simulink model "DBX_model_all"  (R2015a)
settings: Solver=ode2  SolverMode=SingleTasking  StartTime=0.0  StopTime=10  FixedStep=T_sim  RelTol=1e-3
undefined symbols (not defined in the file): A_M, Alpha_unique_rad, as, B_span, Beta_unique_rad, C_D_q, C_l, C_l_delta_a_Asim, C_l_delta_rv_Asim, C_l_p, C_l_r, C_Lift_q, C_m, C_m_q, C_n, C_n_delta_a_Asim, C_n_delta_rv_Asim, C_n_p, C_n_r, C_X, C_Y, C_Y_delta_rv_Asim, C_Y_p, C_Y_r, C_Z, CG, CMA, DBX_aero, DBX_aero_param, delta_elev_unique_rad, DOWN_0, EAST_0, F, g, h_1, h_2, h_3, I_BAC, Initial_Omegas, Initial_Torques, Ion, L_M, Lithium, m, MIL, NORTH_0, P_0, Q_0, R_0, Rotation_sign, Servo_calib, T_sim, U_0, V_0, W_0
libraries: simulink x19, DBX_model x14, aerolibwind2 x12, aerolibasang x9, aerolibadyn x4, aerolibatmos2 x2, powerlib x2, aerolibtransform2 x1, electricdrivelib x1
(part 1 of 3)
settings Model: ExtModeTrigDuration=5000  Creator=DavidTorres  LastModifiedBy=David
settings DataIOCC: LimitDataPoints=off  SaveOutput=off  SignalLogging=off  DSMLogging=off  VisualizeSimOutput=off  SaveTime=off
settings OptimizationCC: InlineParams=on  UseDivisionForNetSlopeComputation=on  UseFloatMulNetSlope=on  InlineInvariantSignals=on  EnhancedBackFolding=on  EfficientFloat2IntCast=on  SimCompilerOptimization=on
settings DebuggingCC: AlgebraicLoopMsg=error  ArtificialAlgebraicLoopMsg=error  SaveWithParameterizedLinksMsg=none  UniqueDataStoreMsg=error  StrictBusMsg=ErrorOnBusTreatedAsVector
settings HardwareCC: ProdLargestAtomicInteger=Long  ProdLargestAtomicFloat=Float  ProdIntDivRoundTo=Zero  ProdEndianess=LittleEndian  ProdHWDeviceType=ARM Compatible->ARM 7  TargetUnknown=on
settings ModelReferenceCC: ModelReferenceNumInstancesAllowed=Single  ModelReferencePassRootInputsByReference=off
settings SimscapeCC: EditingMode=Restricted

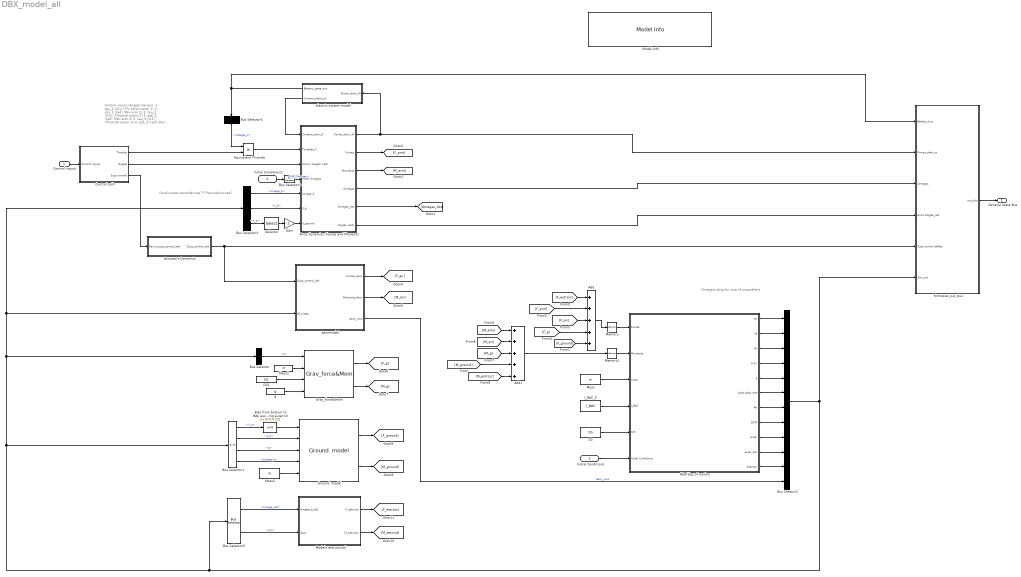
== system DBX_model_all ==
  note: Condiciones atmosfericas???
      | Perturbaciones?
  note: Omegas=Angular rate of proppellers
  note: Control inputs (Angles Servos):
      |
      | 1. tau_1 [0-1] (Thr ottle motor 1)
      | 2. eta_1 (rad)  (Pan arm 1)
      |
      | 3. tau_2 [0-1] (Throttle motor 2)
      | 4. eta_2 (rad)  (Pan arm 2)
      |
      | 5. tau_3 [0-1] (Throttle motor 3)
      | 6. eta_3 (rad)  (Pan arm  3)
      |
      | 7. Rudervator Left (rad)
      | 8. Rudervator Right (rad)
      | 9. Aileron Left (rad)
      | 10. Aielron Right (rad)
  Control Inputs : Inport  PortDimensions=[10,1]
  Initial Conditions : Inport  Port=2  OutDataTypeStr=Bus: slBus1
  6dof Eqs of motion : Subsystem
  Actuators Dynamcis : Subsystem  TreatAsAtomicUnit=on
  Add : Sum  Inputs=+++++
  Add1 : Sum  Inputs=+++++
  Aeromodel : Subsystem  Variant=on  OverrideUsingVariant=DBX_aeroV2_param
  Arms Dynamics: Forces and Moments : Subsystem
  Bias from bottom to BAC assuming euler=0 : Bias  Bias=[0;0;0.25]
  Bus Creator1 : BusCreator  Inputs=12
  Bus Selector : BusSelector  OutputSignals=q
  Bus Selector1 : BusSelector  OutputSignals=X_e,V_b,q,omega_b
  Bus Selector2 : BusSelector  OutputSignals=omega_b,V_b,X_e
  Bus Selector3 : BusSelector  OutputSignals=Init_Omegas
  Bus Selector4 : BusSelector  OutputSignals=Voltage_V
  Bus Selector5 : BusSelector  OutputSignals=omega_dot,A_b
  CG : Constant  Value=CG
  CG1 : Constant  Value=CG
  Control split : Subsystem
  Equivalent Throttle : Product  Inputs=**
  Gain : Gain  Gain=-1
  Grav_force&Mom : DBX_model/Grav_force&Mom
  Ground  model : DBX_model/Ground  model
  I_BAC_0 : Constant  Value=I_BAC
  Initial Conditions1 : InportShadow  Port=2  OutDataTypeStr=Bus: slBus1
  Mass : Constant  Value=m
  Mass1 : Constant  Value=m
  Mass2 : Constant  Value=m
  Memory : Memory  X0=[0,0,0]'  InheritSampleTime=on
  Memory1 : Memory  X0=[0,0,0]'  InheritSampleTime=on
  Model Info : simulink/Model-Wide Utilities/Model Info  Frame=on  DisplayStringWithTags=|  HorizontalTextAlignment=Center  LeftAlignmentValue=0.5  SourceBlockDiagram=DBX_model_all  TagMaxNumber=20
      | Model %<ModelName>
      | 
      | Creado por %<Creator>
      | Modificado el %<LastModificationDate> por %<LastModifiedBy>
      | Version %<ModelVersion>
  Modelo estructural : Subsystem
  Selector : Selector  InputPortWidth=3  Indices=3
  electric system model : Subsystem
  formateo_out_bus : Subsystem
  "g " : Constant  Value=g
  General State Bus : Outport  OutDataTypeStr=Bus: slBus4
  wires:
  Initial Conditions/1 -> 6dof Eqs of motion/6(Initial Conditions)
  6dof Eqs of motion/3(Vb) -> Bus Creator1/3
  6dof Eqs of motion/5(q) -> Bus Creator1/5
  6dof Eqs of motion/2(Ve) -> Bus Creator1/2
  6dof Eqs of motion/6(pdot,qdot,rdot) -> Bus Creator1/6
  6dof Eqs of motion/1(Xe) -> Bus Creator1/1
  6dof Eqs of motion/7(Ab) -> Bus Creator1/7
  6dof Eqs of motion/8(DCM) -> Bus Creator1/8
  6dof Eqs of motion/9(euler) -> Bus Creator1/9
  6dof Eqs of motion/10(euler_dot) -> Bus Creator1/10
  Bus Selector/1 -> Grav_force&Mom/1  "<q>"
  Mass/1 -> 6dof Eqs of motion/3(mass)
  Bus Selector2/1 -> Arms Dynamics: Forces and Moments/5(omega_b)  "<omega_b>"
  Bus Selector2/2 -> Arms Dynamics: Forces and Moments/6(V_b)  "<V_b>"
  Mass1/1 -> Grav_force&Mom/2
  Arms Dynamics: Forces and Moments/5(Omegas_dot) -> [Omegas_dot]
  Initial Conditions1/1 -> Bus Selector3/1
  Bus Selector2/3 -> Selector/1  "<X_e>"
  Selector/1 -> Gain/1
  Gain/1 -> Arms Dynamics: Forces and Moments/7(h_ground)
  Arms Dynamics: Forces and Moments/2(Forces) -> [F_arm]
  Arms Dynamics: Forces and Moments/3(Moments) -> [M_arm]
  Grav_force&Mom/1 -> [F_g]
  [F_arm] -> Add/2
  [F_air] -> Add/3
  [F_g] -> Add/4
  [M_arm] -> Add1/1
  [M_g] -> Add1/3
  [M_air] -> Add1/2
  6dof Eqs of motion/11(Asensor) -> Bus Creator1/11
  Control split/1("Throtles ") -> Equivalent Throttle/2
  Control split/2(Angles) -> Arms Dynamics: Forces and Moments/3(Comm Angles (rad))
  Arms Dynamics: Forces and Moments/4(Omegas) -> formateo_out_bus/3(Omegas)
  Memory/1 -> 6dof Eqs of motion/1(Forces)
  Memory1/1 -> 6dof Eqs of motion/2(Moments)
  CG/1 -> 6dof Eqs of motion/5(CG)
  I_BAC_0/1 -> 6dof Eqs of motion/4(I_BAC)
  Equivalent Throttle/1 -> Arms Dynamics: Forces and Moments/2(Throttles_V)
  Bus Selector4/1 -> Equivalent Throttle/1  "<Voltage_V>"
  6dof Eqs of motion/4(p,q,r) -> Bus Creator1/4
  Arms Dynamics: Forces and Moments/6(Angles (rad)) -> formateo_out_bus/4(Arms Angles_rad)
  Control Inputs/1 -> Control split/1(Control inputs)
  CG1/1 -> Grav_force&Mom/3
  Control split/3(Sups control) -> Actuators Dynamcis/1(Servo_sups_control_rad)
  formateo_out_bus/1(out_bus) -> General State Bus/1
  Bus Selector3/1 -> Arms Dynamics: Forces and Moments/4(Initial Omegas)  "<Init_Omegas>"
  Actuators Dynamcis/1(Sups_control_rad) -> Aeromodel/1(Sups_control_rad), formateo_out_bus/5(Sups control deflec)
  Add/1 -> Memory/1
  Aeromodel/3(Aero_vars) -> Bus Creator1/12  "Aero_vars"
  Add1/1 -> Memory1/1
  Aeromodel/1(Forces_aero) -> [F_air]
  Bus Creator1/1 -> formateo_out_bus/6(Sim_out), Bus Selector5/1, Bus Selector/1, Bus Selector2/1, Aeromodel/2(All_meas), Bus Selector1/1
  Ground  model/1 -> [F_ground]
  Ground  model/2 -> [M_ground]
  Bus Selector1/1 -> Bias from bottom to BAC assuming euler=0/1  "<X_e>"
  Bus Selector1/3 -> Ground  model/3  "<q>"
  Mass2/1 -> Ground  model/5
  Bus Selector1/2 -> Ground  model/2  "<V_b>"
  Bus Selector1/4 -> Ground  model/4  "<omega_b>"
  Bias from bottom to BAC assuming euler=0/1 -> Ground  model/1
  "g "/1 -> Grav_force&Mom/4
  [M_ground] -> Add1/4
  [F_ground] -> Add/5
  Aeromodel/2(Moments_Aero) -> [M_air]
  electric system model/1(Battery_state_bus) -> Bus Selector4/1, formateo_out_bus/1(Battery_bus)
  Arms Dynamics: Forces and Moments/1(Power_drain_W) -> electric system model/1(Power_drain_W), formateo_out_bus/2(Power_drain_w)
  electric system model/2(Current_drains_A) -> Arms Dynamics: Forces and Moments/1(Current_drain_A)
  Bus Selector5/1 -> Modelo estructural/1(omgea_b_dot)  "<omega_dot>"
  Modelo estructural/2(M_estructu) -> [M_estrcut]
  [M_estrcut] -> Add1/5
  Bus Selector5/2 -> Modelo estructural/2(Accs)  "<A_b>"
  Modelo estructural/1(F_estructu) -> [F_estrcut]
  [F_estrcut] -> Add/1
  Grav_force&Mom/2 -> [M_g]

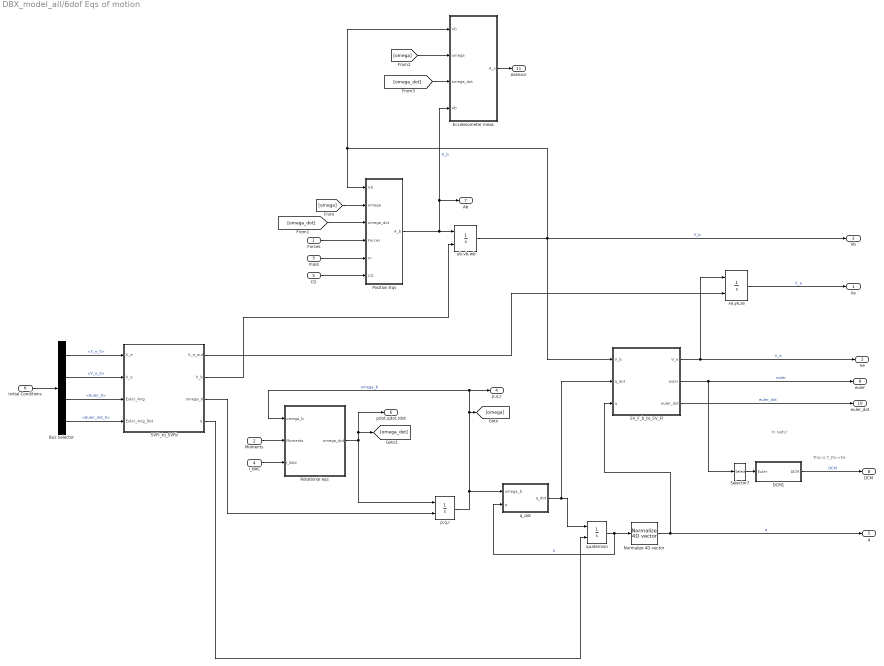
== system DBX_model_all/6dof Eqs of motion ==
  note: In rads!
  note: This is T_Fb->Fe
  Forces : Inport
  Moments : Inport  Port=2
  mass : Inport  Port=3
  I_BAC : Inport  Port=4
  CG : Inport  Port=5
  Initial Conditions : Inport  Port=6
  Bus Selector : BusSelector  OutputSignals=X_e_0,V_e_0,Euler_0,Euler_dot_0
  DCM1 : Subsystem  TreatAsAtomicUnit=on
  Eccelerometer meas : MATLAB Function
  Normalize 4D vector : DBX_model/Normalize 4D vector
  Position Eqs : MATLAB Function
  Rotational eqs : MATLAB Function
  SVFI_to_SVFb : MATLAB Function
  SV_F_b_to_SV_FI : MATLAB Function
  Selector7 : Selector  InputPortWidth=3  Indices=[3 2 1]
  "p,q,r " : Integrator  InitialConditionSource=external  InitialCondition=[P_0,Q_0,R_0]
  q_dot : Subsystem
  quaternion : Integrator  InitialConditionSource=external  InitialCondition=[P_0,Q_0,R_0]
  ub,vb,wb : Integrator  InitialConditionSource=external  InitialCondition=[U_0,V_0,W_0]
  xe,ye,ze : Integrator  InitialConditionSource=external  InitialCondition=[NORTH_0,EAST_0,-DOWN_0]
  Xe : Outport
  Ve : Outport  Port=2
  Vb : Outport  Port=3
  p,q,r : Outport  Port=4
  q : Outport  Port=5
  pdot,qdot,rdot : Outport  Port=6
  Ab : Outport  Port=7
  DCM : Outport  Port=8
  euler : Outport  Port=9
  euler_dot : Outport  Port=10
  Asensor : Outport  Port=11
  wires:
  I_BAC/1 -> Rotational eqs/3(I_BAC)
  mass/1 -> Position Eqs/5(m)
  Forces/1 -> Position Eqs/4(Forces)
  xe,ye,ze/1 -> Xe/1  "X_e"
  ub,vb,wb/1 -> Eccelerometer meas/1(Vb), Position Eqs/1(Vb), Vb/1, SV_F_b_to_SV_FI/1(V_b)  "V_b"
  SV_F_b_to_SV_FI/1(V_e) -> Ve/1, xe,ye,ze/1  "V_e"
  [omega] -> Position Eqs/2(omega)
  [omega_dot] -> Position Eqs/3(omega_dot)
  Position Eqs/1(A_b) -> Eccelerometer meas/4(Ab), Ab/1, ub,vb,wb/1  "A_b"
  CG/1 -> Position Eqs/6(CG)
  Initial Conditions/1 -> Bus Selector/1
  Bus Selector/1 -> SVFI_to_SVFb/1(X_e)  "<X_e_0>"
  Bus Selector/2 -> SVFI_to_SVFb/2(V_e)  "<V_e_0>"
  Bus Selector/3 -> SVFI_to_SVFb/3(Euler_Ang)  "<Euler_0>"
  Bus Selector/4 -> SVFI_to_SVFb/4(Euler_Ang_Dot)  "<Euler_dot_0>"
  SVFI_to_SVFb/2(V_b) -> ub,vb,wb/2
  SVFI_to_SVFb/1(X_e_out) -> xe,ye,ze/2
  SVFI_to_SVFb/3(omega_b) -> "p,q,r "/2
  "p,q,r "/1 -> q_dot/1(omega_b), Rotational eqs/1(omega_b), p,q,r/1, [omega]  "omega_b"
  q_dot/1(q_dot) -> quaternion/1, SV_F_b_to_SV_FI/2(q_dot)
  SVFI_to_SVFb/4(q) -> quaternion/2
  quaternion/1 -> Normalize 4D vector/1, q_dot/2(q)  "q"
  DCM1/1(DCM) -> DCM/1  "DCM"
  SV_F_b_to_SV_FI/3(euler_dot) -> euler_dot/1  "euler_dot"
  Moments/1 -> Rotational eqs/2(Moments)
  Normalize 4D vector/1 -> q/1, SV_F_b_to_SV_FI/3(q)  "q"
  [omega] -> Eccelerometer meas/2(omega)
  [omega_dot] -> Eccelerometer meas/3(omega_dot)
  Eccelerometer meas/1(A_s) -> Asensor/1
  Selector7/1 -> DCM1/1(Euler)
  Rotational eqs/1(omega_dot) -> "p,q,r "/1, pdot,qdot,rdot/1, [omega_dot]
  SV_F_b_to_SV_FI/2(euler) -> Selector7/1, euler/1  "euler"

== system DBX_model_all/Actuators Dynamcis ==
  note: Relaciones no lineales aqui
  note: Control inputs:
      |
      |
      | 7. Rudervator Left (rad)
      | 8. Rudervator Right (rad)
      | 9. Aileron Left (rad)
      | 10. Aielron Right (rad)
  Servo_sups_control_rad : Inport
  Demux : Demux
  Mux2 : Mux
  Servo 1st order : DBX_model/Servo 1st order  Init_def=delta_rv_L_0_servo  Max_rate=6.159  Min_rate=-6.159  Max_defle=deg2rad(25)  Min_def=-deg2rad(25)  RT=0.01
  Servo 1st order1 : DBX_model/Servo 1st order  Init_def=delta_rv_R_0_servo  Max_rate=6.159  Min_rate=-6.159  Max_defle=deg2rad(25)  Min_def=-deg2rad(25)  RT=0.01
  Servo 1st order2 : DBX_model/Servo 1st order  Init_def=delta_a_L_0_servo  Max_rate=6.159  Min_rate=-6.159  Max_defle=deg2rad(25)  Min_def=-deg2rad(25)  RT=0.01
  Servo 1st order3 : DBX_model/Servo 1st order  Init_def=delta_a_R_0_servo  Max_rate=6.159  Min_rate=-6.159  Max_defle=deg2rad(25)  Min_def=-deg2rad(25)  RT=0.01
  Servo2Sup Lin conversion : DBX_model/Servo2Sup Lin conversion  Gain=Servo_calib.Servo4.Pendiente_Sup_Servo  Bias=Servo_calib.Servo4.Sup_rad_0
  Servo2Sup Lin conversion1 : DBX_model/Servo2Sup Lin conversion  Gain=Servo_calib.Servo5.Pendiente_Sup_Servo  Bias=Servo_calib.Servo5.Sup_rad_0
  Servo2Sup Lin conversion2 : DBX_model/Servo2Sup Lin conversion  Gain=Servo_calib.Servo6.Pendiente_Sup_Servo  Bias=Servo_calib.Servo6.Sup_rad_0
  Servo2Sup Lin conversion3 : DBX_model/Servo2Sup Lin conversion  Gain=Servo_calib.Servo7.Pendiente_Sup_Servo  Bias=Servo_calib.Servo7.Sup_rad_0
  Sups_control_rad : Outport
  wires:
  Servo_sups_control_rad/1 -> Demux/1
  Mux2/1 -> Sups_control_rad/1
  Demux/1 -> Servo 1st order/1
  Demux/2 -> Servo 1st order1/1
  Demux/3 -> Servo 1st order2/1
  Demux/4 -> Servo 1st order3/1
  Servo2Sup Lin conversion/1 -> Mux2/1
  Servo2Sup Lin conversion1/1 -> Mux2/2
  Servo2Sup Lin conversion2/1 -> Mux2/3
  Servo2Sup Lin conversion3/1 -> Mux2/4
  Servo 1st order/1 -> Servo2Sup Lin conversion/1
  Servo 1st order1/1 -> Servo2Sup Lin conversion1/1
  Servo 1st order2/1 -> Servo2Sup Lin conversion2/1
  Servo 1st order3/1 -> Servo2Sup Lin conversion3/1

== system DBX_model_all/Aeromodel ==
  note: 1) Add Subsystem or Model blocks as valid variant choices.
      | 2) You cannot connect blocks at this level. At simulation, connectivity is automatically
      | determined, based on the active variant and port name matching.
  Sups_control_rad : Inport
  All_meas : Inport  Port=2
  Aero model V1 : Subsystem  VariantControl=DBX_aeroV1
  Aero model V2 : Subsystem  VariantControl=DBX_aeroV2
  Aero model V2 parametric : Subsystem  VariantControl=DBX_aeroV2_param
  Aero model aerosonde : Subsystem  VariantControl=AeroAerosonde
  Forces_aero : Outport
  Moments_Aero : Outport  Port=2
  Aero_vars : Outport  Port=3

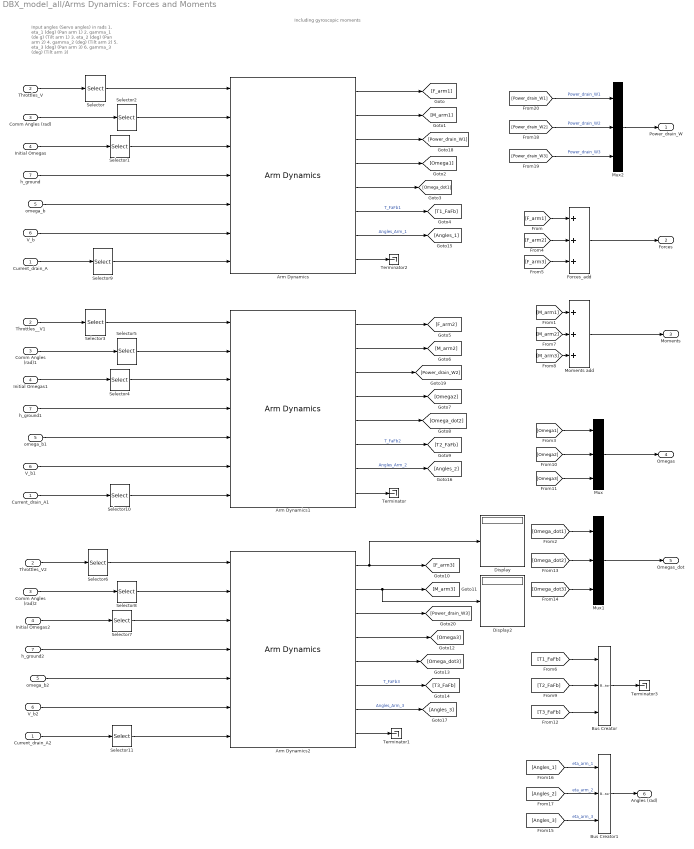
== system DBX_model_all/Arms Dynamics: Forces and Moments ==
  note: Including gyroscopic moments
  note: Input angles (Servo angles)  in rads
      |
      | 1. eta_1 (deg)  (Pan arm 1)
      | 2. gamma_1 (de g)  (Tilt arm 1)
      |
      | 3. eta_2 (deg)  (Pan arm 2)
      | 4. gamma_2 (deg)  (Tilt arm 2)
      |
      | 5. eta_3 (deg)  (Pan arm  3)
      | 6. gamma_3 (deg)  (Tilt arm 3)
  Current_drain_A : Inport
  Throttles_V : Inport  Port=2
  Comm Angles (rad) : Inport  Port=3
  Initial Omegas : Inport  Port=4
  omega_b : Inport  Port=5
  V_b : Inport  Port=6
  h_ground : Inport  Port=7
  Arm Dynamics : DBX_model/Arm Dynamics  arm_num=1  Rot_sign=Rotation_sign(1)  Hub_pos=[1/3*L_M;-A_M/2;h_1]  h_p=hp_1  Gain=[0;1;0]  UpperLimit=deg2rad(10)  LowerLimit=-deg2rad(90)  J_FA=J_FA_1  Inertia_swithc_var=None  Freno_param=Activo  J_T=J_T  tau=Tau_motors  Initi_omega=Initial_Omegas(1)  Init_torque=Initial_Torques(1)  omega_n=40  xi=1.45  init_eta=eta_1_0_servo  Gain_servos=Servo_calib.Servo1.Pendiente_Sup_Servo  Bias=Servo_calib.Servo1.Sup_rad_0
  Arm Dynamics1 : DBX_model/Arm Dynamics  arm_num=2  Rot_sign=Rotation_sign(2)  Hub_pos=[1/3*L_M;A_M/2;h_2]  h_p=hp_2  Gain=[0;1;0]  UpperLimit=deg2rad(10)  LowerLimit=-deg2rad(90)  J_FA=J_FA_2  Inertia_swithc_var=None  Freno_param=Activo  J_T=J_T  tau=Tau_motors  Initi_omega=Initial_Omegas(2)  Init_torque=Initial_Torques(2)  omega_n=40  xi=1.45  init_eta=eta_2_0_servo  Gain_servos=Servo_calib.Servo2.Pendiente_Sup_Servo  Bias=Servo_calib.Servo2.Sup_rad_0
  Arm Dynamics2 : DBX_model/Arm Dynamics  arm_num=3  Rot_sign=Rotation_sign(3)  Hub_pos=[-2/3*L_M;0;h_3]  h_p=hp_3  Gain=[1;0;0]  UpperLimit=deg2rad(60)  LowerLimit=-deg2rad(60)  J_FA=J_FA_3  Inertia_swithc_var=None  Freno_param=Activo  J_T=J_T  tau=Tau_motors  Initi_omega=Initial_Omegas(3)  Init_torque=Initial_Torques(3)  omega_n=40  xi=1.45  init_eta=eta_3_0  Gain_servos=Servo_calib.Servo3.Pendiente_Sup_Servo  Bias=Servo_calib.Servo3.Sup_rad_0
  Bus Creator : BusCreator  Inputs=3
  Bus Creator1 : BusCreator  Inputs=3
  Comm Angles (rad)1 : InportShadow  Port=3
  Comm Angles (rad)2 : InportShadow  Port=3
  Current_drain_A1 : InportShadow
  Current_drain_A2 : InportShadow
  Display : Display
  Display2 : Display
  Forces_add : Sum  Inputs=+++
  Initial Omegas1 : InportShadow  Port=4
  Initial Omegas2 : InportShadow  Port=4
  Moments add : Sum  Inputs=+++
  Mux : Mux  Inputs=3
  Mux1 : Mux  Inputs=3
  Mux2 : Mux  Inputs=3
  Selector : Selector  InputPortWidth=3  Indices=[1]
  Selector1 : Selector  InputPortWidth=3  Indices=[1]
  Selector{3..5,10} (4 alike) : Selector  InputPortWidth=3  Indices=2
  Selector{6..8,11} (4 alike) : Selector  InputPortWidth=3  Indices=3
  Selector2 : Selector  InputPortWidth=3
  Selector9 : Selector  InputPortWidth=3  Indices=[1]
  Terminator{,1..3} (4 alike) : Terminator
  Throttles_V2 : InportShadow  Port=2
  Throttles__V1 : InportShadow  Port=2
  V_b1 : InportShadow  Port=6
  V_b2 : InportShadow  Port=6
  h_ground1 : InportShadow  Port=7
  h_ground2 : InportShadow  Port=7
  omega_b1 : InportShadow  Port=5
  omega_b2 : InportShadow  Port=5
  Power_drain_W : Outport
  Forces : Outport  Port=2
  Moments : Outport  Port=3
  Omegas : Outport  Port=4
  Omegas_dot : Outport  Port=5
  Angles (rad) : Outport  Port=6
  wires:
  Selector1/1 -> Arm Dynamics/3
  Throttles_V/1 -> Selector/1
  Initial Omegas/1 -> Selector1/1
  Selector/1 -> Arm Dynamics/1
  V_b/1 -> Arm Dynamics/6
  Forces_add/1 -> Forces/1
  Moments add/1 -> Moments/1
  Mux/1 -> Omegas/1
  Mux1/1 -> Omegas_dot/1
  h_ground/1 -> Arm Dynamics/4
  Arm Dynamics/1 -> [F_arm1]
  Arm Dynamics/2 -> [M_arm1]
  Arm Dynamics/4 -> [Omega1]
  Arm Dynamics/5 -> [Omega_dot1]
  [F_arm1] -> Forces_add/1
  [M_arm1] -> Moments add/1
  [Omega_dot1] -> Mux1/1
  [Omega1] -> Mux/1
  omega_b/1 -> Arm Dynamics/5
  [F_arm2] -> Forces_add/2
  [F_arm3] -> Forces_add/3
  [Omega2] -> Mux/2
  [Omega3] -> Mux/3
  [Omega_dot2] -> Mux1/2
  [Omega_dot3] -> Mux1/3
  [M_arm3] -> Moments add/3
  [M_arm2] -> Moments add/2
  Selector2/1 -> Arm Dynamics/2
  Comm Angles (rad)/1 -> Selector2/1
  Arm Dynamics/6 -> [T1_FaFb]  "T_FaFb1"
  [T1_FaFb] -> Bus Creator/1
  Selector4/1 -> Arm Dynamics1/3
  Throttles__V1/1 -> Selector3/1
  Initial Omegas1/1 -> Selector4/1
  Selector3/1 -> Arm Dynamics1/1
  V_b1/1 -> Arm Dynamics1/6
  h_ground1/1 -> Arm Dynamics1/4
  Arm Dynamics1/1 -> [F_arm2]
  Arm Dynamics1/2 -> [M_arm2]
  Arm Dynamics1/4 -> [Omega2]
  Arm Dynamics1/5 -> [Omega_dot2]
  omega_b1/1 -> Arm Dynamics1/5
  Selector5/1 -> Arm Dynamics1/2
  Comm Angles (rad)1/1 -> Selector5/1
  Arm Dynamics1/6 -> [T2_FaFb]  "T_FaFb2"
  [T2_FaFb] -> Bus Creator/2
  Selector7/1 -> Arm Dynamics2/3
  Throttles_V2/1 -> Selector6/1
  Initial Omegas2/1 -> Selector7/1
  Selector6/1 -> Arm Dynamics2/1
  V_b2/1 -> Arm Dynamics2/6
  h_ground2/1 -> Arm Dynamics2/4
  Arm Dynamics2/1 -> Display/1, [F_arm3]
  Arm Dynamics2/2 -> Display2/1, [M_arm3]
  Arm Dynamics2/4 -> [Omega3]
  Arm Dynamics2/5 -> [Omega_dot3]
  omega_b2/1 -> Arm Dynamics2/5
  Selector8/1 -> Arm Dynamics2/2
  Comm Angles (rad)2/1 -> Selector8/1
  Arm Dynamics2/6 -> [T3_FaFb]  "T_FaFb3"
  [T3_FaFb] -> Bus Creator/3
  Bus Creator1/1 -> Angles (rad)/1
  [Angles_1] -> Bus Creator1/1  "eta_arm_1"
  [Angles_2] -> Bus Creator1/2  "eta_arm_2"
  [Angles_3] -> Bus Creator1/3  "eta_arm_3"
  Arm Dynamics/7 -> [Angles_1]  "Angles_Arm_1"
  Arm Dynamics1/7 -> [Angles_2]  "Angles_Arm_2"
  Arm Dynamics2/7 -> [Angles_3]  "Angles_Arm_3"
  Arm Dynamics1/8 -> Terminator/1
  Arm Dynamics2/8 -> Terminator1/1
  Arm Dynamics/8 -> Terminator2/1
  Bus Creator/1 -> Terminator3/1
  Current_drain_A/1 -> Selector9/1
  Selector9/1 -> Arm Dynamics/7
  Current_drain_A1/1 -> Selector10/1
  Selector10/1 -> Arm Dynamics1/7
  Current_drain_A2/1 -> Selector11/1
  Selector11/1 -> Arm Dynamics2/7
  Mux2/1 -> Power_drain_W/1
  [Power_drain_W1] -> Mux2/1  "Power_drain_W1"
  [Power_drain_W2] -> Mux2/2  "Power_drain_W2"
  [Power_drain_W3] -> Mux2/3  "Power_drain_W3"
  Arm Dynamics/3 -> [Power_drain_W1]
  Arm Dynamics1/3 -> [Power_drain_W2]
  Arm Dynamics2/3 -> [Power_drain_W3]

== system DBX_model_all/Control split ==
  Control inputs : Inport
  Saturation : Saturate  UpperLimit=1  LowerLimit=0
  Throttles : Selector  InputPortWidth=10  Indices=[1,3,5]
  Throttles1 : Selector  InputPortWidth=10  Indices=[2,4,6]
  Throttles2 : Selector  InputPortWidth=10  Indices=[7:10]
  "Throtles " : Outport
  Angles : Outport  Port=2
  Sups control : Outport  Port=3
  wires:
  Control inputs/1 -> Throttles2/1, Throttles1/1, Throttles/1
  Throttles/1 -> Saturation/1
  Throttles1/1 -> Angles/1
  Saturation/1 -> "Throtles "/1
  Throttles2/1 -> Sups control/1

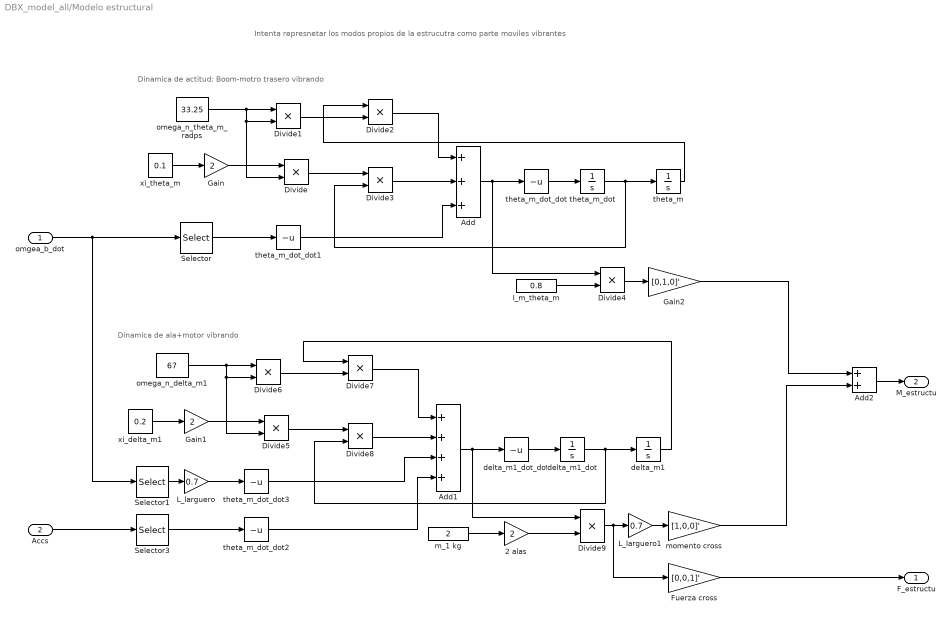
== system DBX_model_all/Modelo estructural ==
  note: Dinamica de actitud: Boom-motro trasero vibrando
  note: Intenta represnetar los modos propios de la estrucutra como parte moviles vibrantes
  note: Dinamica de ala+motor vibrando
  omgea_b_dot : Inport
  Accs : Inport  Port=2
  2 alas : Gain  Gain=2
  Add : Sum  Inputs=+++
  Add1 : Sum  Inputs=++++
  Add2 : Sum
  Divide{,1..9} (10 alike) : Product  Inputs=**
  Fuerza cross : Gain  Gain=[0,0,1]'
  Gain : Gain  Gain=2
  Gain1 : Gain  Gain=2
  Gain2 : Gain  Gain=[0,1,0]'
  I_m_theta_m : Constant  Value=0.8
  L_larguero : Gain  Gain=0.7
  L_larguero1 : Gain  Gain=0.7
  Selector : Selector  InputPortWidth=3  Indices=2
  Selector1 : Selector  InputPortWidth=3
  Selector3 : Selector  InputPortWidth=3  Indices=3
  delta_m1 : Integrator
  delta_m1_dot : Integrator
  delta_m1_dot_dot : UnaryMinus
  m_1 kg : Constant  Value=2
  momento cross : Gain  Gain=[1,0,0]'
  omega_n_delta_m1 : Constant  Value=67
  omega_n_theta_m_radps : Constant  Value=33.25
  theta_m : Integrator
  theta_m_dot : Integrator
  theta_m_dot_dot{,1..3} (4 alike) : UnaryMinus
  xi_delta_m1 : Constant  Value=0.2
  xi_theta_m : Constant  Value=0.1
  F_estructu : Outport
  M_estructu : Outport  Port=2
  wires:
  xi_theta_m/1 -> Gain/1
  Gain/1 -> Divide/1
  omega_n_theta_m_radps/1 -> Divide/2, Divide1/2, Divide1/1
  Divide1/1 -> Divide2/2
  Divide/1 -> Divide3/1
  Divide2/1 -> Add/1
  Divide3/1 -> Add/2
  Selector/1 -> theta_m_dot_dot1/1
  Add/1 -> Divide4/1, theta_m_dot_dot/1
  theta_m_dot_dot/1 -> theta_m_dot/1
  I_m_theta_m/1 -> Divide4/2
  Divide4/1 -> Gain2/1
  theta_m/1 -> Divide2/1
  theta_m_dot/1 -> Divide3/2, theta_m/1
  theta_m_dot_dot1/1 -> Add/3
  xi_delta_m1/1 -> Gain1/1
  Gain1/1 -> Divide5/1
  omega_n_delta_m1/1 -> Divide5/2, Divide6/2, Divide6/1
  Divide6/1 -> Divide7/2
  Divide5/1 -> Divide8/1
  Divide7/1 -> Add1/1
  Divide8/1 -> Add1/2
  omgea_b_dot/1 -> Selector1/1, Selector/1
  Selector1/1 -> L_larguero/1
  Add1/1 -> delta_m1_dot_dot/1, Divide9/1
  delta_m1_dot_dot/1 -> delta_m1_dot/1
  m_1 kg/1 -> 2 alas/1
  delta_m1/1 -> Divide7/1
  delta_m1_dot/1 -> Divide8/2, delta_m1/1
  Add2/1 -> M_estructu/1
  Gain2/1 -> Add2/1
  L_larguero/1 -> theta_m_dot_dot3/1
  Accs/1 -> Selector3/1
  Divide9/1 -> Fuerza cross/1, L_larguero1/1
  2 alas/1 -> Divide9/2
  momento cross/1 -> Add2/2
  Fuerza cross/1 -> F_estructu/1
  theta_m_dot_dot3/1 -> Add1/3
  Selector3/1 -> theta_m_dot_dot2/1
  theta_m_dot_dot2/1 -> Add1/4
  L_larguero1/1 -> momento cross/1

== system DBX_model_all/electric system model ==
  Power_drain_W : Inport
  "29.6 volts, 11.6Ah Li-ion battery " : electricdrivelib/Extra Sources/Battery  BatType=Lithium-Ion  ShowDetailedParameters=off  NomV=29.6  NomQ=11.6  SOC=100  PresetModel=on  MaxQ=11.6  FullV=34.454  Dis_rate=5.0435  R=0.025517  Normal_OP=10.4904  expZone="[31.9794     0.569913]"  current=50  Units=Ampere-hour  Batt_Tr=30
  Bus Creator : BusCreator  Inputs=3
  Bus Selector4 : BusSelector  OutputSignals=Voltage (V)
  Bus to Vector : BusToVector
  Controlled Current Source : powerlib/Electrical Sources/Controlled Current Source  Initialize=on  Source_Type=DC  Amplitude=0  Phase=0  Frequency=0  Measurements=Current
  Demux : Demux  Outputs=3
  Divide : Product  Inputs=/*
  Sum of Elements : Sum  Inputs=+
  initial_current : Memory  InheritSampleTime=on
  powergui : powerlib/powergui  SimulationMode=Discrete  SolverType=Tustin  SampleTime=T_sim  frequency=60  SPID=off  DisableSnubberDevices=off  DisableRonSwitches=off  DisableVfSwitches=off  SwTol=0  DisplayEquations=off  Interpol=off  methode=off  Ts=0  FunctionMessages=off  echomessages=off  HookPort=off  EnableUseOfTLC=off  x0status=blocks  frequencyindice=0  Pbase=100e6  ErrMax=1e-4  Iterations=20  UnitsV=V  UnitsW=W  buscounter=0  RestoreLinks=warning  ResistiveCurrentMeasurement=off  Frange=[0:2:500]  Ylog=off  Xlog=on  ShowGrid=off  save=off  variable=ZData  structure=0  ZoomFFT=on  StartTime=0.0  cycles=1  DisplayStyle=1  fundamental=60  FreqAxis=off  MaxFrequency=1000  frequencyindicesteady=1  RmsSteady=1  display=off
  Battery_state_bus : Outport
  Current_drains_A : Outport  Port=2
  wires:
  "29.6 volts, 11.6Ah Li-ion battery "/1 -> Bus Selector4/1, Bus to Vector/1
  Bus Selector4/1 -> Divide/1  "<Voltage (V)>"
  Divide/1 -> initial_current/1
  Power_drain_W/1 -> Divide/2
  Sum of Elements/1 -> Controlled Current Source/1
  initial_current/1 -> Sum of Elements/1, Current_drains_A/1
  Bus Creator/1 -> Battery_state_bus/1
  Bus to Vector/1 -> Demux/1
  Demux/1 -> Bus Creator/1  "SOC_percent"
  Demux/2 -> Bus Creator/2  "Current_A"
  Demux/3 -> Bus Creator/3  "Voltage_V"
  connections:
  "29.6 volts, 11.6Ah Li-ion battery "/LConn1 -- Controlled Current Source/LConn1
  "29.6 volts, 11.6Ah Li-ion battery "/LConn2 -- Controlled Current Source/RConn1

== system DBX_model_all/formateo_out_bus ==
  Battery_bus : Inport
  Power_drain_w : Inport  Port=2
  Omegas : Inport  Port=3
  Arms Angles_rad : Inport  Port=4
  Sups control deflec : Inport  Port=5
  Sim_out : Inport  Port=6
  Bus Selector3 : BusSelector  OutputSignals=X_e,V_e,V_b,omega_b,q,omega_dot,A_b,DCM,euler,euler_dot,A_s,Aero_vars
  Bus Creator2 : BusCreator  Inputs=17  OutDataTypeStr=Bus: slBus4
  Reshape : Reshape
  out_bus : Outport  OutDataTypeStr=Bus: slBus4
  wires:
  Bus Selector3/6 -> Bus Creator2/6  "<omega_dot>"
  Bus Selector3/9 -> Bus Creator2/9  "<euler>"
  Bus Selector3/4 -> Bus Creator2/4  "<omega_b>"
  Bus Selector3/3 -> Bus Creator2/3  "<V_b>"
  Bus Selector3/7 -> Bus Creator2/7  "<A_b>"
  Bus Selector3/10 -> Bus Creator2/10  "<euler_dot>"
  Bus Selector3/5 -> Bus Creator2/5  "<q>"
  Bus Selector3/8 -> Reshape/1  "<DCM>"
  Bus Selector3/1 -> Bus Creator2/1  "<X_e>"
  Bus Selector3/11 -> Bus Creator2/11  "<A_s>"
  Bus Selector3/2 -> Bus Creator2/2  "<V_e>"
  Sim_out/1 -> Bus Selector3/1
  Reshape/1 -> Bus Creator2/8  "DCM_Vect"
  Omegas/1 -> Bus Creator2/13  "Omegas"
  Arms Angles_rad/1 -> Bus Creator2/14  "Ang_arms_rad"
  Sups control deflec/1 -> Bus Creator2/15  "Sups_control_defl"
  Bus Selector3/12 -> Bus Creator2/12  "<Aero_vars>"
  Battery_bus/1 -> Bus Creator2/16  "Battery_bus"
  Power_drain_w/1 -> Bus Creator2/17  "Power_drain_w"
  Bus Creator2/1 -> out_bus/1

== system DBX_model_all/6dof Eqs of motion/DCM1 ==
  Euler : Inport  PortDimensions=3
  Fcn11 : Fcn  Expr=u(5)*u(4)
  Fcn12 : Fcn  Expr=u(5)*u(1)
  Fcn13 : Fcn  Expr=-u(2)
  Fcn21 : Fcn  Expr=u(3)*u(2)*u(4) - u(6)*u(1)
  Fcn22 : Fcn  Expr=u(3)*u(2)*u(1) + u(6)*u(4)
  Fcn23 : Fcn  Expr=u(3)*u(5)
  Fcn31 : Fcn  Expr=u(6)*u(2)*u(4) + u(3)*u(1)
  Fcn32 : Fcn  Expr=u(6)*u(2)*u(1) - u(3)*u(4)
  Fcn33 : Fcn  Expr=u(6)*u(5)
  Mux : Mux  Inputs=2
  Mux1 : Mux  Inputs=9
  Reshape : Reshape  OutputDimensionality=Customize  OutputDimensions=[3,3]
  sincos : Trigonometry  Operator=sincos
  DCM : Outport  PortDimensions=[3,3]
  wires:
  Fcn33/1 -> Mux1/9
  Fcn32/1 -> Mux1/8
  Fcn23/1 -> Mux1/6
  Fcn22/1 -> Mux1/5
  Fcn31/1 -> Mux1/7
  Fcn21/1 -> Mux1/4
  Fcn13/1 -> Mux1/3
  Fcn12/1 -> Mux1/2
  Fcn11/1 -> Mux1/1
  Mux/1 -> Fcn22/1, Fcn23/1, Fcn31/1, Fcn33/1, Fcn32/1, Fcn21/1, Fcn13/1, Fcn12/1, Fcn11/1
  sincos/2 -> Mux/2
  sincos/1 -> Mux/1
  Reshape/1 -> DCM/1
  Euler/1 -> sincos/1
  Mux1/1 -> Reshape/1

== system DBX_model_all/6dof Eqs of motion/q_dot ==
  note: Both of these methods to compute q_dot are very similar
  omega_b : Inport
  q : Inport  Port=2
  Quaternion_dot : MATLAB Function  TreatAsAtomicUnit=on  VariantControl=Variant
  q_dot : Outport
  wires:
  omega_b/1 -> Quaternion_dot/1(omega_b)  "omega_b"
  q/1 -> Quaternion_dot/2(q)  "q"
  Quaternion_dot/1(q_dot) -> q_dot/1

== system DBX_model_all/Aeromodel/Aero model V1 ==
  Sups_control_rad : Inport
  All_meas : Inport  Port=2
  Aerodynamic Forces and Moments : aerolibadyn/Aerodynamic Forces and Moments   inputAxes=Body  outputForceAxes=Body  outputMomentAxes=Body  S=S_w  b=B_span  cbar=CMA
  Aerodynamics : Subsystem
  Bus Creator : BusCreator
  Bus Selector1 : BusSelector  OutputSignals=V_b,A_b,omega_b,X_e,DCM,V_e
  Constant : Constant  Value=[0,0,0]
  Demux : Demux  Outputs=3
  Gain1 : Gain  Gain=-1
  ISA : MATLAB Function  TreatAsAtomicUnit=on
  Permute Dimensions : PermuteDimensions
  Selector1 : Selector  InputPortWidth=3  Indices=3
  Terminator : Terminator
  Terminator1 : Terminator
  Wind Model : Subsystem
  Forces_aero : Outport
  Moments_Aero : Outport  Port=2
  Aero_vars : Outport  Port=3
  wires:
  All_meas/1 -> Bus Selector1/1
  Sups_control_rad/1 -> Aerodynamics/1(Sups_control_rad)
  Bus Selector1/1 -> Aerodynamics/2(Vb)  "<V_b>"
  Selector1/1 -> Gain1/1
  Bus Selector1/4 -> Selector1/1  "<X_e>"
  Gain1/1 -> ISA/1(altitude), Wind Model/1(Alt (m))
  Bus Selector1/5 -> Wind Model/2(DCM)  "<DCM>"
  Bus Selector1/6 -> Wind Model/3(V_e (m/s))  "<V_e>"
  Wind Model/1(V_wind) -> Aerodynamics/5(V_Wind_b)
  Bus Selector1/2 -> Aerodynamics/3(Vb_dot)  "<A_b>"
  Bus Selector1/3 -> Aerodynamics/4(omega_b)  "<omega_b>"
  Wind Model/2(omega_wind) -> Aerodynamics/6(Wind_omega_b)
  ISA/4(a) -> Aerodynamics/8("a ")
  ISA/1(rho) -> Aerodynamics/7(rho)
  Aerodynamics/2(qbar (pdyn)) -> Bus Creator/1, Aerodynamic Forces and Moments/2  "qbar"
  ISA/2(T) -> Terminator/1
  ISA/3(Ps) -> Terminator1/1
  Constant/1 -> Aerodynamic Forces and Moments/4, Aerodynamic Forces and Moments/3
  Aerodynamics/1(AeroCoeff_b) -> Aerodynamic Forces and Moments/1
  Aerodynamic Forces and Moments/1 -> Forces_aero/1
  Aerodynamic Forces and Moments/2 -> Permute Dimensions/1
  Demux/2 -> Bus Creator/3  "beta"
  Demux/3 -> Bus Creator/4  "alpha"
  Bus Creator/1 -> Aero_vars/1
  Demux/1 -> Bus Creator/2  "TAS"
  Aerodynamics/3(VBetaAlpha) -> Demux/1
  Permute Dimensions/1 -> Moments_Aero/1

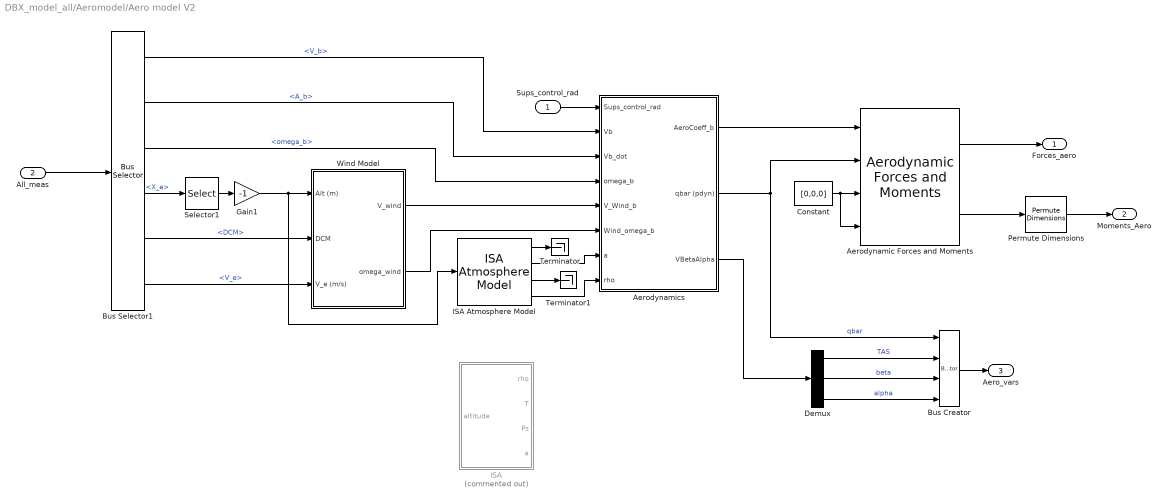
== system DBX_model_all/Aeromodel/Aero model V2 ==
  Sups_control_rad : Inport
  All_meas : Inport  Port=2
  Aerodynamic Forces and Moments : aerolibadyn/Aerodynamic Forces and Moments   inputAxes=Body  outputForceAxes=Body  outputMomentAxes=Body  S=S_w  b=B_span  cbar=CMA
  Aerodynamics : Subsystem
  Bus Creator : BusCreator
  Bus Selector1 : BusSelector  OutputSignals=V_b,A_b,omega_b,X_e,DCM,V_e
  Constant : Constant  Value=[0,0,0]
  Demux : Demux  Outputs=3
  Gain1 : Gain  Gain=-1
  ISA : MATLAB Function  Commented=on  TreatAsAtomicUnit=on
  ISA Atmosphere Model : aerolibatmos2/ISA Atmosphere Model  custom=off  g=9.80665  gamma=1.4  R=287.0531  L=0.0065  h_trop=11000  h_strat=20000  rho0=1.225  P0=101325  T0=288.15  h0=0
  Permute Dimensions : PermuteDimensions
  Selector1 : Selector  InputPortWidth=3  Indices=3
  Terminator : Terminator
  Terminator1 : Terminator
  Wind Model : Subsystem
  Forces_aero : Outport
  Moments_Aero : Outport  Port=2
  Aero_vars : Outport  Port=3
  wires:
  Aerodynamics/3(VBetaAlpha) -> Demux/1
  Demux/1 -> Bus Creator/2  "TAS"
  Bus Creator/1 -> Aero_vars/1
  Demux/3 -> Bus Creator/4  "alpha"
  Demux/2 -> Bus Creator/3  "beta"
  Aerodynamic Forces and Moments/2 -> Permute Dimensions/1
  Aerodynamic Forces and Moments/1 -> Forces_aero/1
  Aerodynamics/1(AeroCoeff_b) -> Aerodynamic Forces and Moments/1
  Constant/1 -> Aerodynamic Forces and Moments/3, Aerodynamic Forces and Moments/4
  ISA Atmosphere Model/3 -> Terminator1/1
  ISA Atmosphere Model/1 -> Terminator/1
  Aerodynamics/2(qbar (pdyn)) -> Aerodynamic Forces and Moments/2, Bus Creator/1  "qbar"
  ISA Atmosphere Model/4 -> Aerodynamics/8(rho)
  ISA Atmosphere Model/2 -> Aerodynamics/7("a ")
  Wind Model/2(omega_wind) -> Aerodynamics/6(Wind_omega_b)
  Bus Selector1/3 -> Aerodynamics/4(omega_b)  "<omega_b>"
  Bus Selector1/2 -> Aerodynamics/3(Vb_dot)  "<A_b>"
  Wind Model/1(V_wind) -> Aerodynamics/5(V_Wind_b)
  Bus Selector1/6 -> Wind Model/3(V_e (m/s))  "<V_e>"
  Bus Selector1/5 -> Wind Model/2(DCM)  "<DCM>"
  Gain1/1 -> ISA Atmosphere Model/1, Wind Model/1(Alt (m))
  Bus Selector1/4 -> Selector1/1  "<X_e>"
  Selector1/1 -> Gain1/1
  Bus Selector1/1 -> Aerodynamics/2(Vb)  "<V_b>"
  Sups_control_rad/1 -> Aerodynamics/1(Sups_control_rad)
  All_meas/1 -> Bus Selector1/1
  Permute Dimensions/1 -> Moments_Aero/1

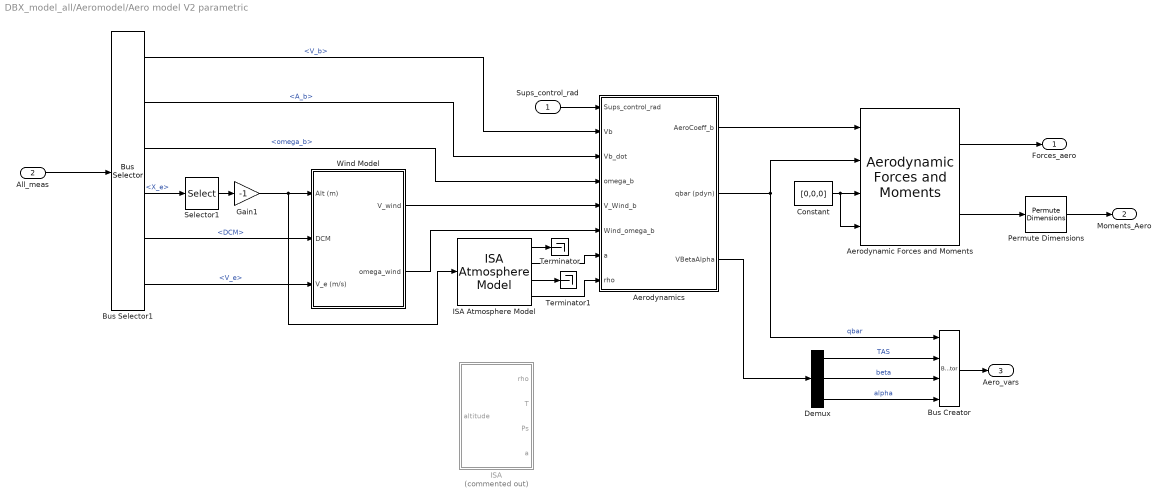
== system DBX_model_all/Aeromodel/Aero model V2 parametric ==
  Sups_control_rad : Inport
  All_meas : Inport  Port=2
  Aerodynamic Forces and Moments : aerolibadyn/Aerodynamic Forces and Moments   inputAxes=Body  outputForceAxes=Body  outputMomentAxes=Body  S=S_w  b=B_span  cbar=CMA
  Aerodynamics : Subsystem
  Bus Creator : BusCreator
  Bus Selector1 : BusSelector  OutputSignals=V_b,A_b,omega_b,X_e,DCM,V_e
  Constant : Constant  Value=[0,0,0]
  Demux : Demux  Outputs=3
  Gain1 : Gain  Gain=-1
  ISA : MATLAB Function  Commented=on  TreatAsAtomicUnit=on
  ISA Atmosphere Model : aerolibatmos2/ISA Atmosphere Model  custom=off  g=9.80665  gamma=1.4  R=287.0531  L=0.0065  h_trop=11000  h_strat=20000  rho0=1.225  P0=101325  T0=288.15  h0=0
  Permute Dimensions : PermuteDimensions
  Selector1 : Selector  InputPortWidth=3  Indices=3
  Terminator : Terminator
  Terminator1 : Terminator
  Wind Model : Subsystem
  Forces_aero : Outport
  Moments_Aero : Outport  Port=2
  Aero_vars : Outport  Port=3
  wires:
  Aerodynamics/3(VBetaAlpha) -> Demux/1
  Demux/1 -> Bus Creator/2  "TAS"
  Bus Creator/1 -> Aero_vars/1
  Demux/3 -> Bus Creator/4  "alpha"
  Demux/2 -> Bus Creator/3  "beta"
  Aerodynamic Forces and Moments/2 -> Permute Dimensions/1
  Aerodynamic Forces and Moments/1 -> Forces_aero/1
  Aerodynamics/1(AeroCoeff_b) -> Aerodynamic Forces and Moments/1
  Constant/1 -> Aerodynamic Forces and Moments/3, Aerodynamic Forces and Moments/4
  ISA Atmosphere Model/3 -> Terminator1/1
  ISA Atmosphere Model/1 -> Terminator/1
  Aerodynamics/2(qbar (pdyn)) -> Aerodynamic Forces and Moments/2, Bus Creator/1  "qbar"
  ISA Atmosphere Model/4 -> Aerodynamics/8(rho)
  ISA Atmosphere Model/2 -> Aerodynamics/7("a ")
  Wind Model/2(omega_wind) -> Aerodynamics/6(Wind_omega_b)
  Bus Selector1/3 -> Aerodynamics/4(omega_b)  "<omega_b>"
  Bus Selector1/2 -> Aerodynamics/3(Vb_dot)  "<A_b>"
  Wind Model/1(V_wind) -> Aerodynamics/5(V_Wind_b)
  Bus Selector1/6 -> Wind Model/3(V_e (m/s))  "<V_e>"
  Bus Selector1/5 -> Wind Model/2(DCM)  "<DCM>"
  Gain1/1 -> ISA Atmosphere Model/1, Wind Model/1(Alt (m))
  Bus Selector1/4 -> Selector1/1  "<X_e>"
  Selector1/1 -> Gain1/1
  Bus Selector1/1 -> Aerodynamics/2(Vb)  "<V_b>"
  Sups_control_rad/1 -> Aerodynamics/1(Sups_control_rad)
  All_meas/1 -> Bus Selector1/1
  Permute Dimensions/1 -> Moments_Aero/1

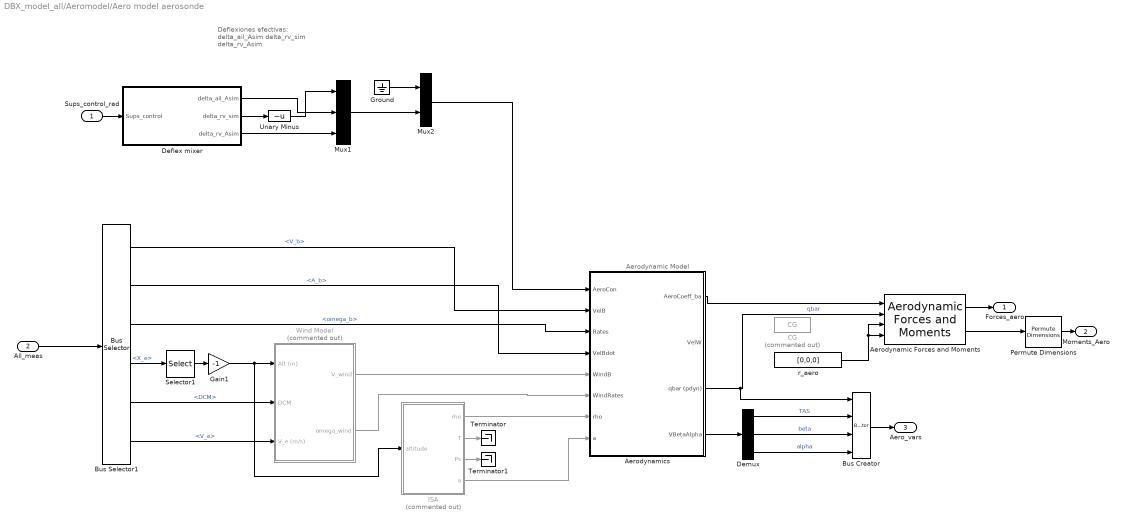
== system DBX_model_all/Aeromodel/Aero model aerosonde ==
  note: Aerodynamic Model
  note: Deflexiones efectivas:
      |
      | delta_ail_Asim
      | delta_rv_sim
      | delta_rv_Asim
  Sups_control_rad : Inport
  All_meas : Inport  Port=2
  Aerodynamic Forces and Moments : aerolibadyn/Aerodynamic Forces and Moments   inputAxes=Body  outputForceAxes=Body  outputMomentAxes=Body  S=S_w  b=B_span  cbar=CMA
  Aerodynamics : Subsystem
  Bus Creator : BusCreator
  Bus Selector1 : BusSelector  OutputSignals=V_b,A_b,omega_b,X_e,DCM,V_e
  CG : Constant  Commented=on  Value=CG
  Deflex mixer : Subsystem  TreatAsAtomicUnit=on
  Demux : Demux  Outputs=3
  Gain1 : Gain  Gain=-1
  Ground : Ground
  ISA : MATLAB Function  Commented=on  TreatAsAtomicUnit=on
  Mux1 : Mux  Inputs=3
  Mux2 : Mux  Inputs=[1,3]
  Permute Dimensions : PermuteDimensions
  Selector1 : Selector  InputPortWidth=3  Indices=3
  Terminator : Terminator
  Terminator1 : Terminator
  Unary Minus : UnaryMinus
  Wind Model : Subsystem  Commented=on
  r_aero : Constant  Value=[0,0,0]
  Forces_aero : Outport
  Moments_Aero : Outport  Port=2
  Aero_vars : Outport  Port=3
  wires:
  Aerodynamic Forces and Moments/2 -> Permute Dimensions/1
  Aerodynamic Forces and Moments/1 -> Forces_aero/1
  r_aero/1 -> Aerodynamic Forces and Moments/3, Aerodynamic Forces and Moments/4
  Aerodynamics/1(AeroCoeff_ba) -> Aerodynamic Forces and Moments/1
  Aerodynamics/3(qbar (pdyn)) -> Bus Creator/1, Aerodynamic Forces and Moments/2  "qbar"
  All_meas/1 -> Bus Selector1/1
  Sups_control_rad/1 -> Deflex mixer/1(Sups_control)
  Bus Selector1/1 -> Aerodynamics/2(VelB)  "<V_b>"
  Selector1/1 -> Gain1/1
  Bus Selector1/4 -> Selector1/1  "<X_e>"
  Gain1/1 -> ISA/1(altitude), Wind Model/1(Alt (m))
  Bus Selector1/5 -> Wind Model/2(DCM)  "<DCM>"
  Bus Selector1/6 -> Wind Model/3(V_e (m/s))  "<V_e>"
  Wind Model/1(V_wind) -> Aerodynamics/5(WindB)
  Bus Selector1/2 -> Aerodynamics/4(VelBdot)  "<A_b>"
  Bus Selector1/3 -> Aerodynamics/3(Rates)  "<omega_b>"
  Wind Model/2(omega_wind) -> Aerodynamics/6(WindRates)
  ISA/4(a) -> Aerodynamics/8("a ")
  ISA/1(rho) -> Aerodynamics/7(rho)
  ISA/2(T) -> Terminator/1
  ISA/3(Ps) -> Terminator1/1
  Mux1/1 -> Mux2/2
  Ground/1 -> Mux2/1
  Deflex mixer/2(delta_rv_sim) -> Unary Minus/1
  Deflex mixer/3(delta_rv_Asim) -> Mux1/3
  Mux2/1 -> Aerodynamics/1(AeroCon)
  Unary Minus/1 -> Mux1/1
  Bus Creator/1 -> Aero_vars/1
  Aerodynamics/4(VBetaAlpha) -> Demux/1
  Demux/1 -> Bus Creator/2  "TAS"
  Demux/2 -> Bus Creator/3  "beta"
  Demux/3 -> Bus Creator/4  "alpha"
  Deflex mixer/1(delta_ail_Asim) -> Mux1/2
  Permute Dimensions/1 -> Moments_Aero/1

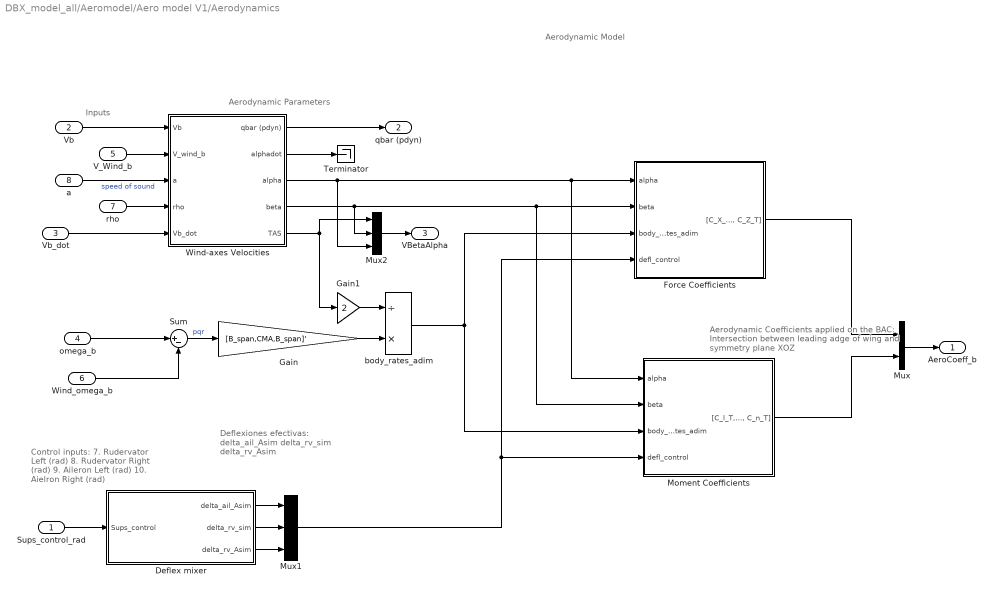
== system DBX_model_all/Aeromodel/Aero model V1/Aerodynamics ==
  note: Deflexiones efectivas:
      |
      | delta_ail_Asim
      | delta_rv_sim
      | delta_rv_Asim
  note: Aerodynamic Model
  note: Aerodynamic Coefficients applied on the BAC:
      |
      | Intersection between leading adge of wing and
      | symmetry plane XOZ
  note: Aerodynamic Parameters
  note: Inputs
  note: Control inputs:
      |
      | 7. Rudervator Left (rad)
      | 8. Rudervator Right (rad)
      | 9. Aileron Left (rad)
      | 10. Aielron Right (rad)
  Sups_control_rad : Inport  PortDimensions=[4 1]
  Vb : Inport  Port=2  PortDimensions=[3 1]
  Vb_dot : Inport  Port=3
  omega_b : Inport  Port=4  PortDimensions=[3 1]
  V_Wind_b : Inport  Port=5  PortDimensions=[3 1]
  Wind_omega_b : Inport  Port=6  PortDimensions=[3 1]
  rho : Inport  Port=7  PortDimensions=1
  "a " : Inport  Port=8  PortDimensions=1
  Deflex mixer : Subsystem  TreatAsAtomicUnit=on
  Force Coefficients : Subsystem
  Gain : Gain  Gain=[B_span,CMA,B_span]'
  Gain1 : Gain  Gain=2
  Moment Coefficients : Subsystem
  Mux : Mux  Inputs=2
  Mux1 : Mux  Inputs=3
  Mux2 : Mux  Inputs=3
  Sum : Sum  Inputs=|+-  SaturateOnIntegerOverflow=on  InputSameDT=on  OutDataTypeStr=Inherit: Same as first input
  Terminator : Terminator
  Wind-axes Velocities : Subsystem
  body_rates_adim : Product  Inputs=/*
  AeroCoeff_b : Outport
  qbar (pdyn) : Outport  Port=2
  VBetaAlpha : Outport  Port=3
  wires:
  Vb_dot/1 -> Wind-axes Velocities/5(Vb_dot)
  V_Wind_b/1 -> Wind-axes Velocities/2(V_wind_b)
  Mux/1 -> AeroCoeff_b/1
  rho/1 -> Wind-axes Velocities/4(rho)
  Vb/1 -> Wind-axes Velocities/1(Vb)
  "a "/1 -> Wind-axes Velocities/3(a)  "speed of sound"
  omega_b/1 -> Sum/1
  Wind_omega_b/1 -> Sum/2
  Sum/1 -> Gain/1  "pqr"
  Sups_control_rad/1 -> Deflex mixer/1(Sups_control)
  Gain/1 -> body_rates_adim/2
  Wind-axes Velocities/5(TAS) -> Gain1/1, Mux2/1
  Gain1/1 -> body_rates_adim/1
  Deflex mixer/1(delta_ail_Asim) -> Mux1/1
  Deflex mixer/2(delta_rv_sim) -> Mux1/2
  Deflex mixer/3(delta_rv_Asim) -> Mux1/3
  Wind-axes Velocities/3(alpha) -> Mux2/3, Force Coefficients/1(alpha), Moment Coefficients/1(alpha)
  body_rates_adim/1 -> Force Coefficients/3(body_rates_adim), Moment Coefficients/3(body_rates_adim)
  Mux1/1 -> Force Coefficients/4(defl_control), Moment Coefficients/4(defl_control)
  Wind-axes Velocities/4(beta) -> Mux2/2, Force Coefficients/2(beta), Moment Coefficients/2(beta)
  Force Coefficients/1("[C_X_T, C_Y_T, C_Z_T]") -> Mux/1
  Moment Coefficients/1("[C_l_T, C_m_T, C_n_T]") -> Mux/2
  Wind-axes Velocities/1(qbar (pdyn)) -> qbar (pdyn)/1
  Wind-axes Velocities/2(alphadot) -> Terminator/1
  Mux2/1 -> VBetaAlpha/1

== system DBX_model_all/Aeromodel/Aero model V1/Wind Model ==
  note: Wind Models
  Alt (m) : Inport
  DCM : Inport  Port=2
  V_e (m/s) : Inport  Port=3
  Dot Product : DotProduct  SaturateOnIntegerOverflow=on  OutDataTypeStr=Inherit: Inherit via internal rule
  Dryden Wind Turbulence Model (Continuous (+q +r)) : aerolibwind2/Dryden Wind Turbulence Model  (Continuous (+q -r))  units=Metric (MKS)  spec=MIL-F-8785C  model=Continuous Von Karman (+q -r)  W20=0  Wdeg=90  TurbProb=2x10^-1  L_high=533.4  Wingspan=B_span  ts=0.02  Seed=[23341 23342 23343 23344]  T_on=on
  Horizontal Wind Model : aerolibwind2/Horizontal Wind Model  units=Metric (MKS)  Vw_source=Internal  Vwind=0  W_source=Internal  Wdeg=-60
  Sum : Sum  Inputs=+++  SaturateOnIntegerOverflow=on  InputSameDT=on  OutDataTypeStr=Inherit: Same as first input
  V : Math  Operator=sqrt  SaturateOnIntegerOverflow=on
  Wind Shear Model : aerolibwind2/Wind Shear Model  units=Metric (MKS)  phase=Category C - Terminal Flight Phase  W_20=0  Wdeg=0
  V_wind : Outport
  omega_wind : Outport  Port=2
  wires:
  V/1 -> Dryden Wind Turbulence Model (Continuous (+q +r))/2
  Dryden Wind Turbulence Model (Continuous (+q +r))/1 -> Sum/3
  V_e (m/s)/1 -> Dot Product/2, Dot Product/1
  Dot Product/1 -> V/1
  Dryden Wind Turbulence Model (Continuous (+q +r))/2 -> omega_wind/1
  Sum/1 -> V_wind/1
  DCM/1 -> Horizontal Wind Model/1, Dryden Wind Turbulence Model (Continuous (+q +r))/3, Wind Shear Model/2
  Alt (m)/1 -> Dryden Wind Turbulence Model (Continuous (+q +r))/1, Wind Shear Model/1
  Horizontal Wind Model/1 -> Sum/2
  Wind Shear Model/1 -> Sum/1

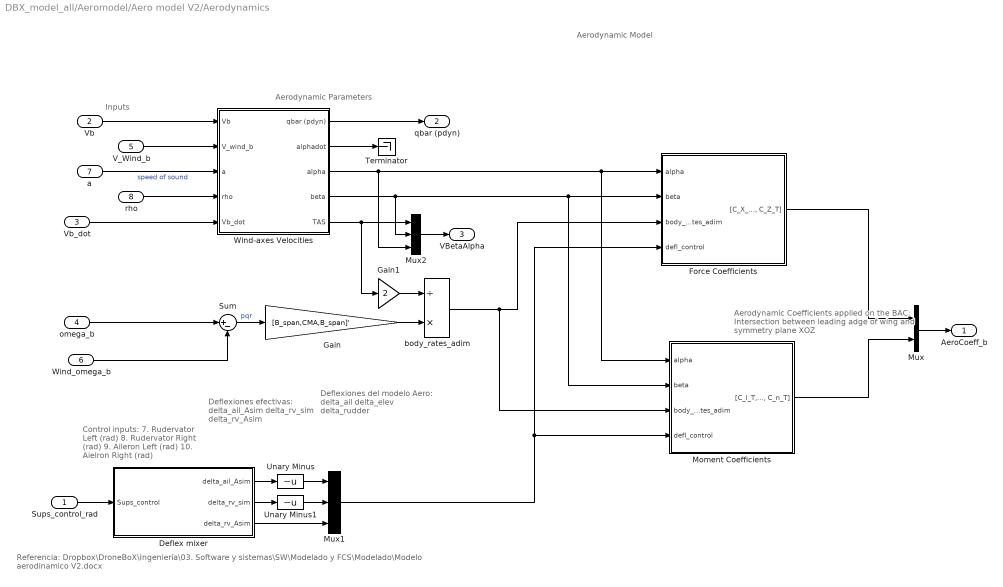
== system DBX_model_all/Aeromodel/Aero model V2/Aerodynamics ==
  note: Referencia:
      | Dropbox\DroneBoX\Ingeniería\03. Software y sistemas\SW\Modelado y FCS\Modelado\Modelo aerodinamico V2.docx
  note: Control inputs:
      |
      | 7. Rudervator Left (rad)
      | 8. Rudervator Right (rad)
      | 9. Aileron Left (rad)
      | 10. Aielron Right (rad)
  note: Inputs
  note: Aerodynamic Parameters
  note: Aerodynamic Coefficients applied on the BAC:
      |
      | Intersection between leading adge of wing and
      | symmetry plane XOZ
  note: Aerodynamic Model
  note: Deflexiones efectivas:
      |
      | delta_ail_Asim
      | delta_rv_sim
      | delta_rv_Asim
  note: Deflexiones del modelo Aero:
      |
      | delta_ail
      | delta_elev
      | delta_rudder
  Sups_control_rad : Inport  PortDimensions=[4 1]
  Vb : Inport  Port=2  PortDimensions=[3 1]
  Vb_dot : Inport  Port=3
  omega_b : Inport  Port=4  PortDimensions=[3 1]
  V_Wind_b : Inport  Port=5  PortDimensions=[3 1]
  Wind_omega_b : Inport  Port=6  PortDimensions=[3 1]
  "a " : Inport  Port=7  PortDimensions=1
  rho : Inport  Port=8  PortDimensions=1
  Deflex mixer : Subsystem  TreatAsAtomicUnit=on
  Force Coefficients : Subsystem
  Gain : Gain  Gain=[B_span,CMA,B_span]'
  Gain1 : Gain  Gain=2
  Moment Coefficients : Subsystem
  Mux : Mux  Inputs=2
  Mux1 : Mux  Inputs=3
  Mux2 : Mux  Inputs=3
  Sum : Sum  Inputs=|+-  SaturateOnIntegerOverflow=on  InputSameDT=on  OutDataTypeStr=Inherit: Same as first input
  Terminator : Terminator
  Unary Minus : UnaryMinus
  Unary Minus1 : UnaryMinus
  Wind-axes Velocities : Subsystem
  body_rates_adim : Product  Inputs=/*
  AeroCoeff_b : Outport
  qbar (pdyn) : Outport  Port=2
  VBetaAlpha : Outport  Port=3
  wires:
  Mux2/1 -> VBetaAlpha/1
  Wind-axes Velocities/2(alphadot) -> Terminator/1
  Wind-axes Velocities/1(qbar (pdyn)) -> qbar (pdyn)/1
  Moment Coefficients/1("[C_l_T, C_m_T, C_n_T]") -> Mux/2
  Force Coefficients/1("[C_X_T, C_Y_T, C_Z_T]") -> Mux/1
  Wind-axes Velocities/4(beta) -> Moment Coefficients/2(beta), Force Coefficients/2(beta), Mux2/2
  Mux1/1 -> Moment Coefficients/4(defl_control), Force Coefficients/4(defl_control)
  body_rates_adim/1 -> Moment Coefficients/3(body_rates_adim), Force Coefficients/3(body_rates_adim)
  Wind-axes Velocities/3(alpha) -> Moment Coefficients/1(alpha), Force Coefficients/1(alpha), Mux2/3
  Deflex mixer/3(delta_rv_Asim) -> Mux1/3
  Deflex mixer/2(delta_rv_sim) -> Unary Minus1/1
  Deflex mixer/1(delta_ail_Asim) -> Unary Minus/1
  Gain1/1 -> body_rates_adim/1
  Wind-axes Velocities/5(TAS) -> Mux2/1, Gain1/1
  Gain/1 -> body_rates_adim/2
  Sups_control_rad/1 -> Deflex mixer/1(Sups_control)
  Sum/1 -> Gain/1  "pqr"
  Wind_omega_b/1 -> Sum/2
  omega_b/1 -> Sum/1
  "a "/1 -> Wind-axes Velocities/3(a)  "speed of sound"
  Vb/1 -> Wind-axes Velocities/1(Vb)
  rho/1 -> Wind-axes Velocities/4(rho)
  Mux/1 -> AeroCoeff_b/1
  V_Wind_b/1 -> Wind-axes Velocities/2(V_wind_b)
  Vb_dot/1 -> Wind-axes Velocities/5(Vb_dot)
  Unary Minus/1 -> Mux1/1
  Unary Minus1/1 -> Mux1/2

== system DBX_model_all/Aeromodel/Aero model V2/Wind Model ==
  note: Wind Models
  Alt (m) : Inport
  DCM : Inport  Port=2
  V_e (m/s) : Inport  Port=3
  Bias : Bias  Bias=eps
  Bias1 : Bias  Bias=eps
  Dot Product : DotProduct  SaturateOnIntegerOverflow=on  OutDataTypeStr=Inherit: Inherit via internal rule
  Dryden Wind Turbulence Model (Continuous (+q +r)) : aerolibwind2/Dryden Wind Turbulence Model  (Continuous (+q -r))  units=Metric (MKS)  spec=MIL-F-8785C  model=Continuous Von Karman (+q -r)  W20=0  Wdeg=90  TurbProb=2x10^-1  L_high=533.4  Wingspan=B_span  ts=T_sim  Seed=[23341 23342 23343 23344]  T_on=on
  Horizontal Wind Model : aerolibwind2/Horizontal Wind Model  units=Metric (MKS)  Vw_source=Internal  Vwind=0  W_source=Internal  Wdeg=-60
  Sum : Sum  Inputs=+++  SaturateOnIntegerOverflow=on  InputSameDT=on  OutDataTypeStr=Inherit: Same as first input
  V : Math  Operator=sqrt  SaturateOnIntegerOverflow=on
  Wind Shear Model : aerolibwind2/Wind Shear Model  units=Metric (MKS)  phase=Category C - Terminal Flight Phase  W_20=0  Wdeg=0
  V_wind : Outport
  omega_wind : Outport  Port=2
  wires:
  Wind Shear Model/1 -> Sum/1
  Horizontal Wind Model/1 -> Sum/2
  Alt (m)/1 -> Dryden Wind Turbulence Model (Continuous (+q +r))/1, Wind Shear Model/1
  DCM/1 -> Horizontal Wind Model/1, Dryden Wind Turbulence Model (Continuous (+q +r))/3, Wind Shear Model/2
  Sum/1 -> Bias1/1
  Dryden Wind Turbulence Model (Continuous (+q +r))/2 -> omega_wind/1
  Dot Product/1 -> V/1
  V_e (m/s)/1 -> Dot Product/2, Dot Product/1
  Dryden Wind Turbulence Model (Continuous (+q +r))/1 -> Sum/3
  V/1 -> Bias/1
  Bias/1 -> Dryden Wind Turbulence Model (Continuous (+q +r))/2
  Bias1/1 -> V_wind/1

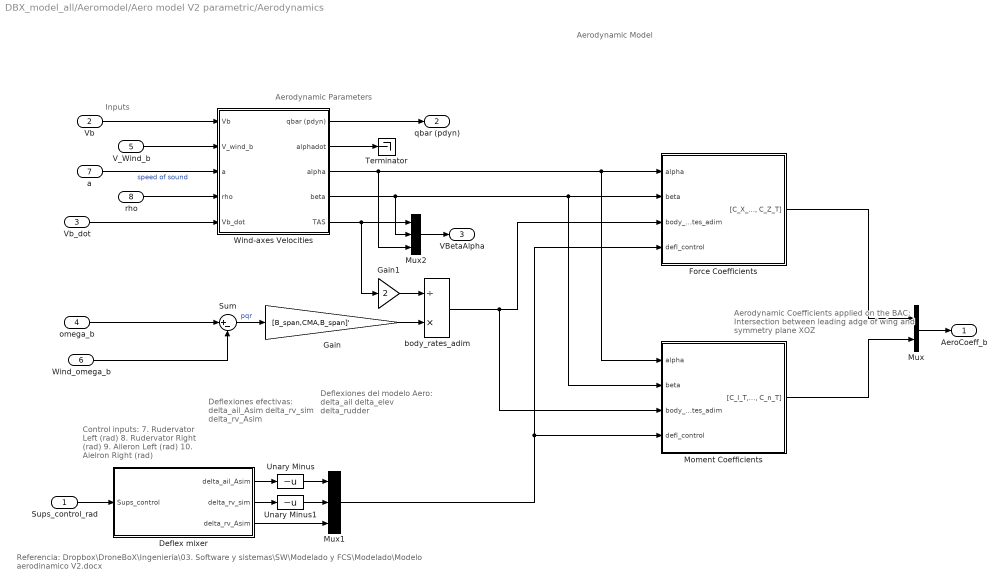
== system DBX_model_all/Aeromodel/Aero model V2 parametric/Aerodynamics ==
  note: Referencia:
      | Dropbox\DroneBoX\Ingeniería\03. Software y sistemas\SW\Modelado y FCS\Modelado\Modelo aerodinamico V2.docx
  note: Control inputs:
      |
      | 7. Rudervator Left (rad)
      | 8. Rudervator Right (rad)
      | 9. Aileron Left (rad)
      | 10. Aielron Right (rad)
  note: Inputs
  note: Aerodynamic Parameters
  note: Aerodynamic Coefficients applied on the BAC:
      |
      | Intersection between leading adge of wing and
      | symmetry plane XOZ
  note: Aerodynamic Model
  note: Deflexiones efectivas:
      |
      | delta_ail_Asim
      | delta_rv_sim
      | delta_rv_Asim
  note: Deflexiones del modelo Aero:
      |
      | delta_ail
      | delta_elev
      | delta_rudder
  Sups_control_rad : Inport  PortDimensions=[4 1]
  Vb : Inport  Port=2  PortDimensions=[3 1]
  Vb_dot : Inport  Port=3
  omega_b : Inport  Port=4  PortDimensions=[3 1]
  V_Wind_b : Inport  Port=5  PortDimensions=[3 1]
  Wind_omega_b : Inport  Port=6  PortDimensions=[3 1]
  "a " : Inport  Port=7  PortDimensions=1
  rho : Inport  Port=8  PortDimensions=1
  Deflex mixer : Subsystem  TreatAsAtomicUnit=on
  Force Coefficients : Subsystem  TreatAsAtomicUnit=on
  Gain : Gain  Gain=[B_span,CMA,B_span]'
  Gain1 : Gain  Gain=2
  Moment Coefficients : Subsystem  TreatAsAtomicUnit=on
  Mux : Mux  Inputs=2
  Mux1 : Mux  Inputs=3
  Mux2 : Mux  Inputs=3
  Sum : Sum  Inputs=|+-  SaturateOnIntegerOverflow=on  InputSameDT=on  OutDataTypeStr=Inherit: Same as first input
  Terminator : Terminator
  Unary Minus : UnaryMinus
  Unary Minus1 : UnaryMinus
  Wind-axes Velocities : Subsystem
  body_rates_adim : Product  Inputs=/*
  AeroCoeff_b : Outport
  qbar (pdyn) : Outport  Port=2
  VBetaAlpha : Outport  Port=3
  wires:
  Mux2/1 -> VBetaAlpha/1
  Wind-axes Velocities/2(alphadot) -> Terminator/1
  Wind-axes Velocities/1(qbar (pdyn)) -> qbar (pdyn)/1
  Moment Coefficients/1("[C_l_T, C_m_T, C_n_T]") -> Mux/2
  Force Coefficients/1("[C_X_T, C_Y_T, C_Z_T]") -> Mux/1
  Wind-axes Velocities/4(beta) -> Moment Coefficients/2(beta), Force Coefficients/2(beta), Mux2/2
  Mux1/1 -> Moment Coefficients/4(defl_control), Force Coefficients/4(defl_control)
  body_rates_adim/1 -> Moment Coefficients/3(body_rates_adim), Force Coefficients/3(body_rates_adim)
  Wind-axes Velocities/3(alpha) -> Moment Coefficients/1(alpha), Force Coefficients/1(alpha), Mux2/3
  Deflex mixer/3(delta_rv_Asim) -> Mux1/3
  Deflex mixer/2(delta_rv_sim) -> Unary Minus1/1
  Deflex mixer/1(delta_ail_Asim) -> Unary Minus/1
  Gain1/1 -> body_rates_adim/1
  Wind-axes Velocities/5(TAS) -> Mux2/1, Gain1/1
  Gain/1 -> body_rates_adim/2
  Sups_control_rad/1 -> Deflex mixer/1(Sups_control)
  Sum/1 -> Gain/1  "pqr"
  Wind_omega_b/1 -> Sum/2
  omega_b/1 -> Sum/1
  "a "/1 -> Wind-axes Velocities/3(a)  "speed of sound"
  Vb/1 -> Wind-axes Velocities/1(Vb)
  rho/1 -> Wind-axes Velocities/4(rho)
  Mux/1 -> AeroCoeff_b/1
  V_Wind_b/1 -> Wind-axes Velocities/2(V_wind_b)
  Vb_dot/1 -> Wind-axes Velocities/5(Vb_dot)
  Unary Minus/1 -> Mux1/1
  Unary Minus1/1 -> Mux1/2
